simulink model "ITMBS_LEGO_Emergency_PB"  (R2023a)
settings: Solver=FixedStepDiscrete  StartTime=0.0  StopTime=20  FixedStep=0.05  RelTol=1e-3
undefined symbols (not defined in the file): sigbuilder_block
libraries: legoev3lib x3
settings Model: Creator=3w07  LastModifiedBy=manis
settings OptimizationCC: ReuseModelBlockBuffer=off

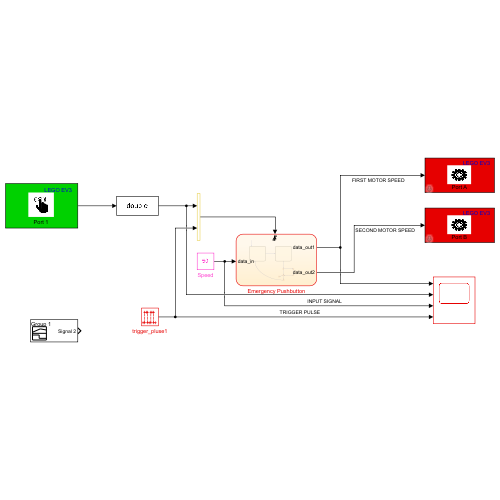
[thumbnail: Simulink's stored preview of the top-level diagram]
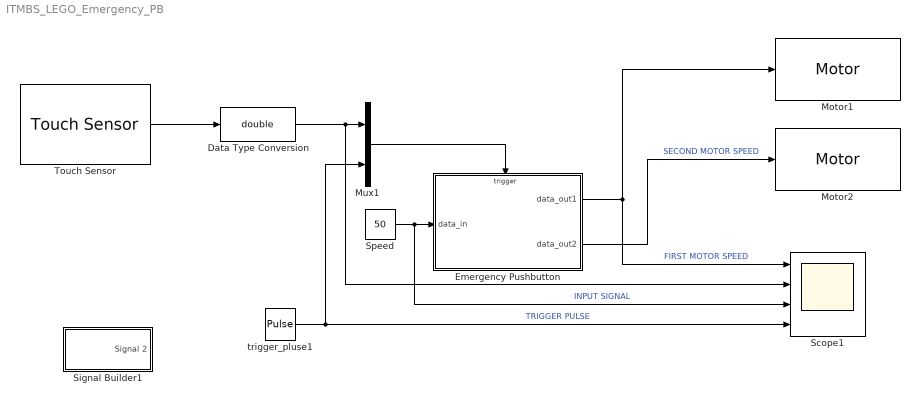
== system ITMBS_LEGO_Emergency_PB ==
  Data Type Conversion : DataTypeConversion  OutDataTypeStr=double  SaturateOnIntegerOverflow=off  RndMeth=Floor
  Emergency Pushbutton : Stateflow chart  TreatAsAtomicUnit=on
  Motor1 : legoev3lib/Motor  sportNumber=A  sstopAction=Brake
  Motor2 : legoev3lib/Motor  sportNumber=B  sstopAction=Brake
  Mux1 : Mux  Inputs=2
  Scope1 : Scope  NumInputPorts=4
  Signal Builder1 : Subsystem  Tag=STV Subsys  LoadFcn=sigbuilder_block('load');  StartFcn=sigbuilder_block('start');  StopFcn=sigbuilder_block('stop');  ClipboardFcn=sigbuilder_block('clipboard');  mask(Sigbuilder block){tuvar=[0:10]}
      mask help: Simulink:masks:SigbuilderBlock_MD
      mask init:
      | if ~strcmp(get_param(bdroot(gcbh),'SimulationStatus'),'stopped') tuvar = sigbuilder_block('maskInit'); end
      settings: CopyFcn=sigbuilder_block('copy');  DeleteFcn=sigbuilder_block('delete');  ModelCloseFcn=sigbuilder_block('modelClose');  PreSaveFcn=sigbuilder_block('preSave');  PauseFcn=sigbuilder_block('pause');  ContinueFcn=sigbuilder_block('continue');  NameChangeFcn=sigbuilder_block('namechange');  OpenFcn=sigbuilder_block('open',[5.4 36 1141.2 516.6 ]);  CloseFcn=sigbuilder_block('close');
      mask Display: plot(0, 0, 100, 100,[2, 2, 32, 32, 2], [68, 8, 8, 68, 68],[32, 2], [38, 38], [32, 19, 2],[53, 60, 44], [32, 17, 17, 2],[16, 16, 31, 31]);txt = getActiveGroup(gcbh);text(2, 100, txt,'verticalAlignment', 'top');
  Speed : Constant  Value=50
  Touch Sensor : legoev3lib/Touch Sensor  portNumber=1  sampleTime=0.1
  trigger_pluse1 : DiscretePulseGenerator  Period=10  PulseWidth=2  SampleTime=0.05
  wires:
  Mux1/1 -> Emergency Pushbutton/Trigger
  Emergency Pushbutton/1(data_out1) -> Scope1/1, Motor1/1  "FIRST MOTOR SPEED"
  trigger_pluse1/1 -> Scope1/4, Mux1/2  "TRIGGER PULSE"
  Data Type Conversion/1 -> Scope1/2, Mux1/1
  Speed/1 -> Emergency Pushbutton/1(data_in), Scope1/3  "INPUT SIGNAL"
  Touch Sensor/1 -> Data Type Conversion/1
  Emergency Pushbutton/2(data_out2) -> Motor2/1  "SECOND MOTOR SPEED"

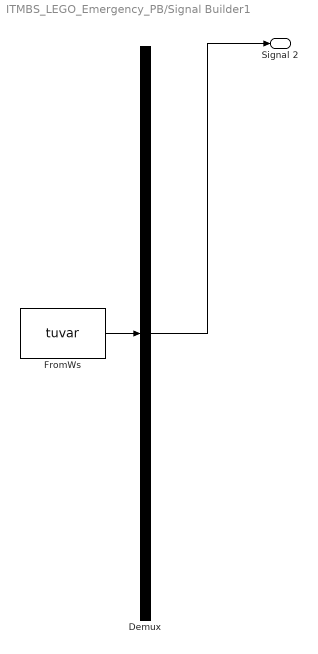
== system ITMBS_LEGO_Emergency_PB/Signal Builder1 ==
  Demux : Demux  Tag=STV Demux  Outputs=1
      settings: DisplayOption=none
  FromWs : FromWorkspace  Tag=STV FromWs  VariableName=tuvar
      SigBuilderData=|
      | common.afterFinalStr = 'Extrapolate'
      | common.sampleTime = 0
      | dataSet.timeRange = [0 20]
      | dataSet.name = 'Group 1'
      | sbobj.Groups.Name = 'Group 1'
      | sbobj.Groups.Signals.Name = 'Signal 2'
      | sbobj.Groups.Signals.XData = [0 4.19 4.19 4.28 4.28 6.036 6.301 6.301 6.401 6.401 6.499 6.499 6.601 6.601 20]
      | sbobj.Groups.Signals.YData = [0 0 1 1 0 0 0 0.995 0.995 0 0 0.995 0.995 0 0]
      | sbobj.Groups.TimeRange = [0 20]
  Signal 2 : Outport  Tag=STV Outport
  wires:
  FromWs/1 -> Demux/1
  Demux/1 -> Signal 2/1

== stateflow chart ITMBS_LEGO_Emergency_PB/Emergency Pushbutton ==
  state state_1
    data_out1=data_in
    data_out2=data_in
  state state_2
    data_out1=0;
    data_out2=0;
    entry:
    counter=0;
  (default) -> state_1
  state_1 -> state_2 : pb_event
  (junction 93) -> state_1 : [counter==2]
  state_2 -> (junction 97) : %pb_event
  (junction 97) -> (junction 98) [order 1] : [pb_event]
  (junction 97) -> (junction 99) [order 2]
  (junction 98) -> (junction 107) : {counter=counter+1}
  (junction 107) -> (junction 99)
  (junction 99) -> (junction 104) [order 2]
  (junction 99) -> (junction 93) [order 1]
  data: data_in input; data_out1 output; counter local; data_out2 output
  events: pb_event input RISING_EDGE_EVENT; event input RISING_EDGE_EVENT
